simulink subsystem "CantileverCartesianRobotSubsystem"  (R2024a)
settings: Solver=VariableStepAuto  StartTime=0.0  StopTime=10.0  RelTol=1e-3
model mask{DOF=3DOF, configAxis=XYZ, heightColumn=0.4, widthColumn=0.05, positionColumn1=[-0.5,-0.5,0], positionColumn2=[0.5,-0.5,0], systemGuideX=Rail-block, strokeXMax=1, widthGuideX=0.05, diaScrewX=0.05, widthXMount=0.1, typeInertiaGuideX=Calculate from Geometry, densityGuideX=2700, massGuideX=0.1, COMGuideX=[0 0 0], MOIGuideX=[0.01 0.01 0.01], POIGuideX=[0 0 0], typeInertiaCarriageX=Calculate from Geometry, densityCarriageX=2700, massCarriageX=0.1, COMCarriageX=[0 0 0], MOICarriageX=[0.01 0.01 0.01], POICarriageX=[0 0 0], colorGuideX=[0.7 0.6 0.4], colorCarriageX=[0.5 0.5 0.9], systemGuideY=Rail-block, strokeYMax=1, widthGuideY=0.05, diaScrewY=0.05, widthYMount=0.05, typeInertiaGuideY=Calculate from Geometry, densityGuideY=2700, massGuideY=0.1, COMGuideY=[0 0 0], MOIGuideY=[0.01 0.01 0.01], POIGuideY=[0 0 0], typeInertiaCarriageY=Calculate from Geometry, densityCarriageY=2700, massCarriageY=0.1, COMCarriageY=[0 0 0], MOICarriageY=[0.01 0.01 0.01], POICarriageY=[0 0 0], colorGuideY=[0.7 0.6 0.4], colorCarriageY=[0.5 0.5 0.9], systemGuideZ=Rail-block, strokeZMax=1, widthGuideZ=0.05, diaScrewZ=0.05, shiftZAxisDown=015, widthZMount=0.05, typeInertiaGuideZ=Calculate from Geometry, densityGuideZ=2700, massGuideZ=0.1, COMGuideZ=[0 0 0], MOIGuideZ=[0.01 0.01 0.01], POIGuideZ=[0 0 0], typeInertiaCarriageZ=Calculate from Geometry, densityCarriageZ=2700, massCarriageZ=0.1, COMCarriageZ=[0 0 0], MOICarriageZ=[0.01 0.01 0.01], POICarriageZ=[0 0 0], colorGuideZ=[0.7 0.6 0.4], colorCarriageZ=[0.5 0.5 0.9]}
  mask prompts: DOF "Degrees of freedom"; configAxis "Axis configurations"; heightColumn "Column height (m)"; widthColumn "Column width (m)"; positionColumn1 "Column 1 position (m)"; positionColumn2 "Column 2 position (m)"; systemGuideX "Guide system"; strokeXMax "Maximum stroke (m)"; widthGuideX "Guide width (m)"; diaScrewX "Screw diameter (m)"; widthXMount "Mount width (m)"; typeInertiaGuideX "Inertia type"; densityGuideX "Density (kg/m^3)"; massGuideX "Mass (kg)"; COMGuideX "Center of mass (m)"; MOIGuideX "Moments of inertia (kg*m^2)"; POIGuideX "Products of inertia (kg*m^2)"; typeInertiaCarriageX "Inertia type"; densityCarriageX "Density (kg/m^3)"; massCarriageX "Mass (kg)"; COMCarriageX "Center of mass (m)"; MOICarriageX "Moments of inertia (kg*m^2)"; POICarriageX "Products of inertia (kg*m^2)"; colorGuideX "Linear guide color"; colorCarriageX "Carriage color"; systemGuideY "Guide system"; strokeYMax "Maximum stroke (m)"; widthGuideY "Guide width (m)"; diaScrewY "Screw diameter (m)"; widthYMount "Mount width (m)"; typeInertiaGuideY "Inertia type"; densityGuideY "Density (kg/m^3)"; massGuideY "Mass (kg)"; COMGuideY "Center of mass (m)"; MOIGuideY "Moments of inertia (kg*m^2)"; POIGuideY "Products of inertia (kg*m^2)"; typeInertiaCarriageY "Inertia type"; densityCarriageY "Density (kg/m^3)"; massCarriageY "Mass (kg)"; COMCarriageY "Center of mass (m)"; MOICarriageY "Moments of inertia (kg*m^2)"; POICarriageY "Products of inertia (kg*m^2)"; colorGuideY "Linear guide color"; colorCarriageY "Carriage color"; systemGuideZ "Guide system"; strokeZMax "Maximum stroke (m)"; widthGuideZ "Guide width (m)"; diaScrewZ "Screw diameter (m)"; shiftZAxisDown "Downward shift of Z-axis (m)"; widthZMount "Mount width (m)"; typeInertiaGuideZ "Inertia type"; densityGuideZ "Density (kg/m^3)"; massGuideZ "Mass (kg)"; COMGuideZ "Center of mass (m)"; MOIGuideZ "Moments of inertia (kg*m^2)"; POIGuideZ "Products of inertia (kg*m^2)"; typeInertiaCarriageZ "Inertia type"; densityCarriageZ "Density (kg/m^3)"; massCarriageZ "Mass (kg)"; COMCarriageZ "Center of mass (m)"; MOICarriageZ "Moments of inertia (kg*m^2)"; POICarriageZ "Products of inertia (kg*m^2)"; colorGuideZ "Linear guide color"; colorCarriageZ "Carriage color"
undefined symbols (not defined in the file): CartesianRobot, X, Y, Z
libraries: sm_lib x99, CartesianLib x44, nesl_utility x41
(part 2 of 4)

== system CantileverCartesianRobotSubsystem/CantileverCartesianRobotVariant/XY Cartesian/Structure1 ==
  Column1 : CartesianLib/Column  lengthColumn=heightColumn  widthColumn=widthColumn  typeInertiaColumn=Calculate from Geometry  densityColumn=7780  massColumn=1  CMColumn=[0 0 0]  MOIColumn=[1 1 1]  POIColumn=[0 0 0]  colorColumn=[0.8 0.2 0.2]
  Column2 : CartesianLib/Column  lengthColumn=heightColumn  widthColumn=widthColumn  typeInertiaColumn=Calculate from Geometry  densityColumn=7780  massColumn=1  CMColumn=[0 0 0]  MOIColumn=[1 1 1]  POIColumn=[0 0 0]  colorColumn=[0.8 0.2 0.2]
  Rigid Transform1 : sm_lib/Frames and Transforms/Rigid Transform  RotationMethod=None  FollAlignAxisA=+X  BaseAlignAxisA=+Y  FollAlignAxisB=+Y  BaseAlignAxisB=+Z  RotationStandardAxis=+Z  RotationAngle=0  RotationAngleUnits=deg  RotationArbitraryAxis=[0 0 1]  RotationSequenceAxes=FollowerAxes  RotationSequence=XYX  RotationSequenceAngles=[0 0 0]  RotationSequenceAnglesUnits=deg  RotationMatrix=[1 0 0;0 1 0;0 0 1]  Quaternion=[1 0 0 0]  TranslationMethod=Cartesian  TranslationCartesianOffset=positionColumn1  TranslationCartesianOffsetUnits=m  TranslationStandardAxis=+Z  TranslationStandardOffset=0  TranslationStandardOffsetUnits=m  TranslationROffset=0  TranslationROffsetUnits=m  TranslationThetaOffset=0  TranslationThetaOffsetUnits=deg  TranslationZOffset=0  TranslationZOffsetUnits=m
  Rigid Transform2 : sm_lib/Frames and Transforms/Rigid Transform  RotationMethod=None  FollAlignAxisA=+X  BaseAlignAxisA=+Y  FollAlignAxisB=+Y  BaseAlignAxisB=+Z  RotationStandardAxis=+Z  RotationAngle=0  RotationAngleUnits=deg  RotationArbitraryAxis=[0 0 1]  RotationSequenceAxes=FollowerAxes  RotationSequence=XYX  RotationSequenceAngles=[0 0 0]  RotationSequenceAnglesUnits=deg  RotationMatrix=[1 0 0;0 1 0;0 0 1]  Quaternion=[1 0 0 0]  TranslationMethod=Cartesian  TranslationCartesianOffset=positionColumn2  TranslationCartesianOffsetUnits=m  TranslationStandardAxis=+Z  TranslationStandardOffset=0  TranslationStandardOffsetUnits=m  TranslationROffset=0  TranslationROffsetUnits=m  TranslationThetaOffset=0  TranslationThetaOffsetUnits=deg  TranslationZOffset=0  TranslationZOffsetUnits=m
  Weld Joint : sm_lib/Joints/Weld Joint  JointMode=Normal  CompositeWrenchDir=FollowerOnBase  CompositeWrenchFrame=BaseFrame  SenseConstraintForce=off  SenseConstraintTorque=off  SenseTotalForce=off  SenseTotalTorque=off
  Weld Joint1 : sm_lib/Joints/Weld Joint  JointMode=Normal  CompositeWrenchDir=FollowerOnBase  CompositeWrenchFrame=BaseFrame  SenseConstraintForce=off  SenseConstraintTorque=off  SenseTotalForce=off  SenseTotalTorque=off
  XMount1 : CartesianLib/Mount  typeMount=Plate mount  widthMount=widthXMount  angleMount=45  angleRotate=0  typeInertiaMount=Calculate from Geometry  densityMount=7780  massMount=0.1  CMMount=[0 0 0]  MOIMount=[1 1 1]  POIMount=[0 0 0]  colorMount=[0.35 0.25 0.25]
  XMount2 : CartesianLib/Mount  typeMount=Plate mount  widthMount=widthXMount  angleMount=45  angleRotate=0  typeInertiaMount=Calculate from Geometry  densityMount=7780  massMount=0.1  CMMount=[0 0 0]  MOIMount=[1 1 1]  POIMount=[0 0 0]  colorMount=[0.35 0.25 0.25]
  F1 : PMIOPort  Side=Left
  B : PMIOPort  Port=2  Side=Right
  F2 : PMIOPort  Port=3  Side=Left
  connections:
  Weld Joint1/RConn1 -- Column2/RConn1
  Rigid Transform1/RConn1 -- Weld Joint/LConn1
  Rigid Transform2/RConn1 -- Weld Joint1/LConn1
  B/RConn1 -- Rigid Transform2/LConn1 -- Rigid Transform1/LConn1
  F2/RConn1 -- XMount2/LConn1
  XMount2/RConn1 -- Column2/LConn1
  Column1/LConn1 -- XMount1/RConn1
  XMount1/LConn1 -- F1/RConn1
  Weld Joint/RConn1 -- Column1/RConn1

== system CantileverCartesianRobotSubsystem/CantileverCartesianRobotVariant/XY Cartesian/Subsystem ==
  note: Dummy ZS signals
  Constant : Constant  Value=0
  Constant1 : Constant  Value=0
  Constant2 : Constant  Value=0
  Bus Element Out : Outport  PortName=ZS  Element=Zp (m)
  BusElementOut : Outport  PortName=ZS  Element=Zv (m/s)
  BusElementOut1 : Outport  PortName=ZS  Element=Za (m^2/s)
  wires:
  Constant/1 -> Bus Element Out/1
  Constant1/1 -> BusElementOut/1
  Constant2/1 -> BusElementOut1/1

== system CantileverCartesianRobotSubsystem/CantileverCartesianRobotVariant/XY Cartesian/Subsystem1 ==
  note: Dummy RS signals
  Constant : Constant  Value=0
  Constant1 : Constant  Value=0
  Bus Element Out : Outport  PortName=RS  Element=q (rad)
  BusElementOut : Outport  PortName=RS  Element=w (rad/s)
  wires:
  Constant/1 -> Bus Element Out/1
  Constant1/1 -> BusElementOut/1

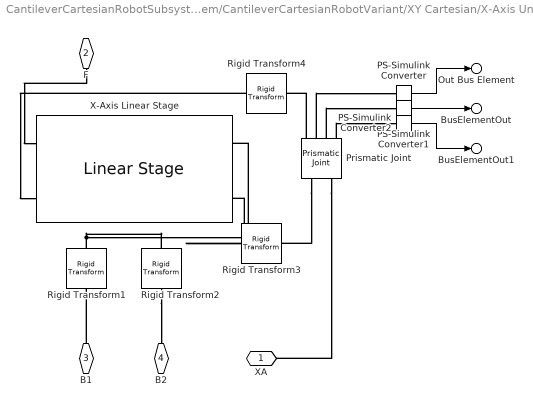
== system CantileverCartesianRobotSubsystem/CantileverCartesianRobotVariant/XY Cartesian/X-Axis Unit ==
  PS-Simulink Converter : nesl_utility/PS-Simulink Converter  PhysicalDomain=network_engine_domain  SubClassName=ps_output  LeftPortType=input  RightPortType=output  PseudoPeriodic=off  Frequencies=[]  VectorFormat=inherit  Unit=inherit  AffineConversion=off
  PS-Simulink Converter1 : nesl_utility/PS-Simulink Converter  PhysicalDomain=network_engine_domain  SubClassName=ps_output  LeftPortType=input  RightPortType=output  PseudoPeriodic=off  Frequencies=[]  VectorFormat=inherit  Unit=inherit  AffineConversion=off
  PS-Simulink Converter2 : nesl_utility/PS-Simulink Converter  PhysicalDomain=network_engine_domain  SubClassName=ps_output  LeftPortType=input  RightPortType=output  PseudoPeriodic=off  Frequencies=[]  VectorFormat=inherit  Unit=inherit  AffineConversion=off
  Prismatic Joint : sm_lib/Joints/Prismatic Joint  JointMode=Normal  CompositeWrenchDir=FollowerOnBase  CompositeWrenchFrame=BaseFrame  SenseConstraintForce=off  SenseConstraintTorque=off  SenseTotalForce=off  SenseTotalTorque=off  PositionTargetSpecify=off  PositionTargetPriority=High  PositionTargetValue=0  PositionTargetValueUnits=m  VelocityTargetSpecify=off  VelocityTargetPriority=High  VelocityTargetValue=0  VelocityTargetValueUnits=m/s  EquilibriumPosition=0  EquilibriumPositionUnits=m  SpringStiffness=0  SpringStiffnessUnits=N/m  DampingCoefficient=0  DampingCoefficientUnits=N/(m/s)  LowerLimitSpecify=on  LowerLimitBound=-0.5*strokeXMax  LowerLimitBoundUnits=m  LowerLimitStiffness=1e6  LowerLimitStiffnessUnits=N/m  LowerLimitDamping=1e3  LowerLimitDampingUnits=N/(m/s)  LowerLimitTransitionRegionWidth=1e-4  LowerLimitTransitionRegionWidthUnits=m  UpperLimitSpecify=on  UpperLimitBound=0.5*strokeXMax  UpperLimitBoundUnits=m  UpperLimitStiffness=1e6  UpperLimitStiffnessUnits=N/m  UpperLimitDamping=1e3  UpperLimitDampingUnits=N/(m/s)  UpperLimitTransitionRegionWidth=1e-4  UpperLimitTransitionRegionWidthUnits=m  TorqueActuationMode=InputTorque  MotionActuationMode=ComputedMotion  SensePosition=on  SenseVelocity=on  SenseAcceleration=on  SenseTorqueForce=off  SenseLowerLimitTorqueForce=off  SenseUpperLimitTorqueForce=off
  Rigid Transform1 : sm_lib/Frames and Transforms/Rigid Transform  RotationMethod=None  FollAlignAxisA=+X  BaseAlignAxisA=+Y  FollAlignAxisB=+Y  BaseAlignAxisB=+Z  RotationStandardAxis=+Z  RotationAngle=0  RotationAngleUnits=deg  RotationArbitraryAxis=[0 0 1]  RotationSequenceAxes=FollowerAxes  RotationSequence=XYX  RotationSequenceAngles=[0 0 0]  RotationSequenceAnglesUnits=deg  RotationMatrix=[1 0 0;0 1 0;0 0 1]  Quaternion=[1 0 0 0]  TranslationMethod=StandardAxis  TranslationCartesianOffset=[-positionColumn1(1) 0 0]  TranslationCartesianOffsetUnits=m  TranslationStandardAxis=+X  TranslationStandardOffset=-positionColumn1(1)  TranslationStandardOffsetUnits=m  TranslationROffset=0  TranslationROffsetUnits=m  TranslationThetaOffset=0  TranslationThetaOffsetUnits=deg  TranslationZOffset=0  TranslationZOffsetUnits=m
  Rigid Transform2 : sm_lib/Frames and Transforms/Rigid Transform  RotationMethod=None  FollAlignAxisA=+X  BaseAlignAxisA=+Y  FollAlignAxisB=+Y  BaseAlignAxisB=+Z  RotationStandardAxis=+Z  RotationAngle=0  RotationAngleUnits=deg  RotationArbitraryAxis=[0 0 1]  RotationSequenceAxes=FollowerAxes  RotationSequence=XYX  RotationSequenceAngles=[0 0 0]  RotationSequenceAnglesUnits=deg  RotationMatrix=[1 0 0;0 1 0;0 0 1]  Quaternion=[1 0 0 0]  TranslationMethod=StandardAxis  TranslationCartesianOffset=[-positionColumn2(1) 0 0]  TranslationCartesianOffsetUnits=m  TranslationStandardAxis=+X  TranslationStandardOffset=-positionColumn2(1)  TranslationStandardOffsetUnits=m  TranslationROffset=0  TranslationROffsetUnits=m  TranslationThetaOffset=0  TranslationThetaOffsetUnits=deg  TranslationZOffset=0  TranslationZOffsetUnits=m
  Rigid Transform3 : sm_lib/Frames and Transforms/Rigid Transform  RotationMethod=StandardAxis  FollAlignAxisA=+X  BaseAlignAxisA=+Y  FollAlignAxisB=+Y  BaseAlignAxisB=+Z  RotationStandardAxis=+Y  RotationAngle=90  RotationAngleUnits=deg  RotationArbitraryAxis=[0 0 1]  RotationSequenceAxes=FollowerAxes  RotationSequence=XYX  RotationSequenceAngles=[0 0 0]  RotationSequenceAnglesUnits=deg  RotationMatrix=[1 0 0;0 1 0;0 0 1]  Quaternion=[1 0 0 0]  TranslationMethod=None  TranslationCartesianOffset=[0 0 0]  TranslationCartesianOffsetUnits=m  TranslationStandardAxis=+Z  TranslationStandardOffset=0  TranslationStandardOffsetUnits=m  TranslationROffset=0  TranslationROffsetUnits=m  TranslationThetaOffset=0  TranslationThetaOffsetUnits=deg  TranslationZOffset=0  TranslationZOffsetUnits=m
  Rigid Transform4 : sm_lib/Frames and Transforms/Rigid Transform  RotationMethod=StandardAxis  FollAlignAxisA=+X  BaseAlignAxisA=+Y  FollAlignAxisB=+Y  BaseAlignAxisB=+Z  RotationStandardAxis=+Y  RotationAngle=-90  RotationAngleUnits=deg  RotationArbitraryAxis=[0 0 1]  RotationSequenceAxes=FollowerAxes  RotationSequence=XYX  RotationSequenceAngles=[0 0 0]  RotationSequenceAnglesUnits=deg  RotationMatrix=[1 0 0;0 1 0;0 0 1]  Quaternion=[1 0 0 0]  TranslationMethod=None  TranslationCartesianOffset=[0 0 0]  TranslationCartesianOffsetUnits=m  TranslationStandardAxis=+Z  TranslationStandardOffset=0  TranslationStandardOffsetUnits=m  TranslationROffset=0  TranslationROffsetUnits=m  TranslationThetaOffset=0  TranslationThetaOffsetUnits=deg  TranslationZOffset=0  TranslationZOffsetUnits=m
  X-Axis Linear Stage : CartesianLib/Linear Stage  systemGuide=Rail-block  axisGuide=X-axis  stroke=1  widthRail=0.05  diaScrew=0.05  typeInertiaGuide=Calculate from Geometry  densityGuide=2700  massGuide=0.1  CMGuide=[0 0 0]  MOIGuide=[0.01 0.01 0.01]  POIGuide=[0 0 0]  typeInertiaCarriage=Calculate from Geometry  densityCarriage=2700  massCarriage=0.1  CMCarriage=[0 0 0]  MOICarriage=[0.01 0.01 0.01]  POICarriage=[0 0 0]  colorGuide=colorGuideX  colorCarriage=colorCarriageX
  XA : PMIOPort  Side=Left
  F : PMIOPort  Port=2  Side=Left
  B1 : PMIOPort  Port=3  Side=Right
  B2 : PMIOPort  Port=4  Side=Right
  Out Bus Element : Outport  PortName=XS  Element=Xp (m)
  BusElementOut : Outport  PortName=XS  Element=Xv (m/s)
  BusElementOut1 : Outport  PortName=XS  Element=Xa (m^2/s)
  wires:
  PS-Simulink Converter2/1 -> BusElementOut1/1
  PS-Simulink Converter1/1 -> BusElementOut/1
  PS-Simulink Converter/1 -> Out Bus Element/1
  connections:
  Prismatic Joint/RConn4 -- PS-Simulink Converter2/LConn1
  Prismatic Joint/RConn3 -- PS-Simulink Converter1/LConn1
  Prismatic Joint/RConn2 -- PS-Simulink Converter/LConn1
  Rigid Transform2/LConn1 -- B2/RConn1
  Rigid Transform3/LConn1 -- X-Axis Linear Stage/RConn2
  X-Axis Linear Stage/RConn1 -- Rigid Transform2/RConn1 -- Rigid Transform1/RConn1
  Prismatic Joint/LConn1 -- Rigid Transform3/RConn1
  F/RConn1 -- X-Axis Linear Stage/LConn1
  Prismatic Joint/RConn1 -- Rigid Transform4/LConn1
  B1/RConn1 -- Rigid Transform1/LConn1
  Prismatic Joint/LConn2 -- XA/RConn1
  Rigid Transform4/RConn1 -- X-Axis Linear Stage/LConn2

== system CantileverCartesianRobotSubsystem/CantileverCartesianRobotVariant/XY Cartesian/Y-Axis Unit ==
  PS-Simulink Converter : nesl_utility/PS-Simulink Converter  PhysicalDomain=network_engine_domain  SubClassName=ps_output  LeftPortType=input  RightPortType=output  PseudoPeriodic=off  Frequencies=[]  VectorFormat=inherit  Unit=inherit  AffineConversion=off
  PS-Simulink Converter1 : nesl_utility/PS-Simulink Converter  PhysicalDomain=network_engine_domain  SubClassName=ps_output  LeftPortType=input  RightPortType=output  PseudoPeriodic=off  Frequencies=[]  VectorFormat=inherit  Unit=inherit  AffineConversion=off
  PS-Simulink Converter2 : nesl_utility/PS-Simulink Converter  PhysicalDomain=network_engine_domain  SubClassName=ps_output  LeftPortType=input  RightPortType=output  PseudoPeriodic=off  Frequencies=[]  VectorFormat=inherit  Unit=inherit  AffineConversion=off
  Prismatic Joint2 : sm_lib/Joints/Prismatic Joint  JointMode=Normal  CompositeWrenchDir=FollowerOnBase  CompositeWrenchFrame=BaseFrame  SenseConstraintForce=off  SenseConstraintTorque=off  SenseTotalForce=off  SenseTotalTorque=off  PositionTargetSpecify=off  PositionTargetPriority=High  PositionTargetValue=0  PositionTargetValueUnits=m  VelocityTargetSpecify=off  VelocityTargetPriority=High  VelocityTargetValue=0  VelocityTargetValueUnits=m/s  EquilibriumPosition=0  EquilibriumPositionUnits=m  SpringStiffness=0  SpringStiffnessUnits=N/m  DampingCoefficient=0  DampingCoefficientUnits=N/(m/s)  LowerLimitSpecify=on  LowerLimitBound=-0.5*strokeYMax  LowerLimitBoundUnits=m  LowerLimitStiffness=1e6  LowerLimitStiffnessUnits=N/m  LowerLimitDamping=1e3  LowerLimitDampingUnits=N/(m/s)  LowerLimitTransitionRegionWidth=1e-4  LowerLimitTransitionRegionWidthUnits=m  UpperLimitSpecify=on  UpperLimitBound=0.5*strokeYMax  UpperLimitBoundUnits=m  UpperLimitStiffness=1e6  UpperLimitStiffnessUnits=N/m  UpperLimitDamping=1e3  UpperLimitDampingUnits=N/(m/s)  UpperLimitTransitionRegionWidth=1e-4  UpperLimitTransitionRegionWidthUnits=m  TorqueActuationMode=InputTorque  MotionActuationMode=ComputedMotion  SensePosition=on  SenseVelocity=on  SenseAcceleration=on  SenseTorqueForce=off  SenseLowerLimitTorqueForce=off  SenseUpperLimitTorqueForce=off
  Rigid Transform1 : sm_lib/Frames and Transforms/Rigid Transform  RotationMethod=None  FollAlignAxisA=+X  BaseAlignAxisA=+Y  FollAlignAxisB=+Y  BaseAlignAxisB=+Z  RotationStandardAxis=+Z  RotationAngle=0  RotationAngleUnits=deg  RotationArbitraryAxis=[0 0 1]  RotationSequenceAxes=BaseAxes  RotationSequence=XYZ  RotationSequenceAngles=[0 0 0]  RotationSequenceAnglesUnits=deg  RotationMatrix=[1 0 0;0 1 0;0 0 1]  Quaternion=[1 0 0 0]  TranslationMethod=StandardAxis  TranslationCartesianOffset=[0 0 0]  TranslationCartesianOffsetUnits=m  TranslationStandardAxis=+Y  TranslationStandardOffset=-positionColumn1(2)  TranslationStandardOffsetUnits=m  TranslationROffset=0  TranslationROffsetUnits=m  TranslationThetaOffset=0  TranslationThetaOffsetUnits=deg  TranslationZOffset=0  TranslationZOffsetUnits=m
  Rigid Transform3 : sm_lib/Frames and Transforms/Rigid Transform  RotationMethod=StandardAxis  FollAlignAxisA=+X  BaseAlignAxisA=+Y  FollAlignAxisB=+Y  BaseAlignAxisB=+Z  RotationStandardAxis=+X  RotationAngle=-90  RotationAngleUnits=deg  RotationArbitraryAxis=[0 0 1]  RotationSequenceAxes=FollowerAxes  RotationSequence=XYX  RotationSequenceAngles=[0 0 0]  RotationSequenceAnglesUnits=deg  RotationMatrix=[1 0 0;0 1 0;0 0 1]  Quaternion=[1 0 0 0]  TranslationMethod=None  TranslationCartesianOffset=[0 0 0]  TranslationCartesianOffsetUnits=m  TranslationStandardAxis=+Z  TranslationStandardOffset=0  TranslationStandardOffsetUnits=m  TranslationROffset=0  TranslationROffsetUnits=m  TranslationThetaOffset=0  TranslationThetaOffsetUnits=deg  TranslationZOffset=0  TranslationZOffsetUnits=m
  Rigid Transform4 : sm_lib/Frames and Transforms/Rigid Transform  RotationMethod=StandardAxis  FollAlignAxisA=+X  BaseAlignAxisA=+Y  FollAlignAxisB=+Y  BaseAlignAxisB=+Z  RotationStandardAxis=+X  RotationAngle=90  RotationAngleUnits=deg  RotationArbitraryAxis=[0 0 1]  RotationSequenceAxes=FollowerAxes  RotationSequence=XYX  RotationSequenceAngles=[0 0 0]  RotationSequenceAnglesUnits=deg  RotationMatrix=[1 0 0;0 1 0;0 0 1]  Quaternion=[1 0 0 0]  TranslationMethod=None  TranslationCartesianOffset=[0 0 0]  TranslationCartesianOffsetUnits=m  TranslationStandardAxis=+Z  TranslationStandardOffset=0  TranslationStandardOffsetUnits=m  TranslationROffset=0  TranslationROffsetUnits=m  TranslationThetaOffset=0  TranslationThetaOffsetUnits=deg  TranslationZOffset=0  TranslationZOffsetUnits=m
  Y-Axis Linear Stage : CartesianLib/Linear Stage  systemGuide=Rail-block  axisGuide=Y-axis  stroke=1  widthRail=0.05  diaScrew=0.05  typeInertiaGuide=Calculate from Geometry  densityGuide=2700  massGuide=0.1  CMGuide=[0 0 0]  MOIGuide=[0.01 0.01 0.01]  POIGuide=[0 0 0]  typeInertiaCarriage=Calculate from Geometry  densityCarriage=2700  massCarriage=0.1  CMCarriage=[0 0 0]  MOICarriage=[0.01 0.01 0.01]  POICarriage=[0 0 0]  colorGuide=colorGuideY  colorCarriage=colorCarriageY
  YA : PMIOPort  Side=Left
  F : PMIOPort  Port=2  Side=Left
  B : PMIOPort  Port=3  Side=Right
  Out Bus Element : Outport  PortName=YS  Element=Yp (m)
  BusElementOut : Outport  PortName=YS  Element=Yv (m/s)
  BusElementOut1 : Outport  PortName=YS  Element=Ya (m^2/s)
  wires:
  PS-Simulink Converter2/1 -> BusElementOut1/1
  PS-Simulink Converter1/1 -> BusElementOut/1
  PS-Simulink Converter/1 -> Out Bus Element/1
  connections:
  Prismatic Joint2/RConn2 -- PS-Simulink Converter/LConn1
  PS-Simulink Converter2/LConn1 -- Prismatic Joint2/RConn4
  Prismatic Joint2/RConn3 -- PS-Simulink Converter1/LConn1
  F/RConn1 -- Y-Axis Linear Stage/LConn1
  Rigid Transform1/LConn1 -- B/RConn1
  Prismatic Joint2/LConn2 -- YA/RConn1
  Rigid Transform1/RConn1 -- Y-Axis Linear Stage/RConn1
  Prismatic Joint2/RConn1 -- Rigid Transform4/LConn1
  Rigid Transform3/LConn1 -- Y-Axis Linear Stage/RConn2
  Rigid Transform4/RConn1 -- Y-Axis Linear Stage/LConn2
  Prismatic Joint2/LConn1 -- Rigid Transform3/RConn1

== system CantileverCartesianRobotSubsystem/CantileverCartesianRobotVariant/XYZ Cartesian/Structure1 ==
  Column1 : CartesianLib/Column  lengthColumn=heightColumn  widthColumn=widthColumn  typeInertiaColumn=Calculate from Geometry  densityColumn=7780  massColumn=1  CMColumn=[0 0 0]  MOIColumn=[1 1 1]  POIColumn=[0 0 0]  colorColumn=[0.8 0.2 0.2]
  Column2 : CartesianLib/Column  lengthColumn=heightColumn  widthColumn=widthColumn  typeInertiaColumn=Calculate from Geometry  densityColumn=7780  massColumn=1  CMColumn=[0 0 0]  MOIColumn=[1 1 1]  POIColumn=[0 0 0]  colorColumn=[0.8 0.2 0.2]
  Rigid Transform1 : sm_lib/Frames and Transforms/Rigid Transform  RotationMethod=None  FollAlignAxisA=+X  BaseAlignAxisA=+Y  FollAlignAxisB=+Y  BaseAlignAxisB=+Z  RotationStandardAxis=+Z  RotationAngle=0  RotationAngleUnits=deg  RotationArbitraryAxis=[0 0 1]  RotationSequenceAxes=FollowerAxes  RotationSequence=XYX  RotationSequenceAngles=[0 0 0]  RotationSequenceAnglesUnits=deg  RotationMatrix=[1 0 0;0 1 0;0 0 1]  Quaternion=[1 0 0 0]  TranslationMethod=Cartesian  TranslationCartesianOffset=positionColumn1  TranslationCartesianOffsetUnits=m  TranslationStandardAxis=+Z  TranslationStandardOffset=0  TranslationStandardOffsetUnits=m  TranslationROffset=0  TranslationROffsetUnits=m  TranslationThetaOffset=0  TranslationThetaOffsetUnits=deg  TranslationZOffset=0  TranslationZOffsetUnits=m
  Rigid Transform2 : sm_lib/Frames and Transforms/Rigid Transform  RotationMethod=None  FollAlignAxisA=+X  BaseAlignAxisA=+Y  FollAlignAxisB=+Y  BaseAlignAxisB=+Z  RotationStandardAxis=+Z  RotationAngle=0  RotationAngleUnits=deg  RotationArbitraryAxis=[0 0 1]  RotationSequenceAxes=FollowerAxes  RotationSequence=XYX  RotationSequenceAngles=[0 0 0]  RotationSequenceAnglesUnits=deg  RotationMatrix=[1 0 0;0 1 0;0 0 1]  Quaternion=[1 0 0 0]  TranslationMethod=Cartesian  TranslationCartesianOffset=positionColumn2  TranslationCartesianOffsetUnits=m  TranslationStandardAxis=+Z  TranslationStandardOffset=0  TranslationStandardOffsetUnits=m  TranslationROffset=0  TranslationROffsetUnits=m  TranslationThetaOffset=0  TranslationThetaOffsetUnits=deg  TranslationZOffset=0  TranslationZOffsetUnits=m
  Weld Joint : sm_lib/Joints/Weld Joint  JointMode=Normal  CompositeWrenchDir=FollowerOnBase  CompositeWrenchFrame=BaseFrame  SenseConstraintForce=off  SenseConstraintTorque=off  SenseTotalForce=off  SenseTotalTorque=off
  Weld Joint1 : sm_lib/Joints/Weld Joint  JointMode=Normal  CompositeWrenchDir=FollowerOnBase  CompositeWrenchFrame=BaseFrame  SenseConstraintForce=off  SenseConstraintTorque=off  SenseTotalForce=off  SenseTotalTorque=off
  XMount1 : CartesianLib/Mount  typeMount=Plate mount  widthMount=widthXMount  angleMount=45  angleRotate=0  typeInertiaMount=Calculate from Geometry  densityMount=7780  massMount=0.1  CMMount=[0 0 0]  MOIMount=[1 1 1]  POIMount=[0 0 0]  colorMount=[0.35 0.25 0.25]
  XMount2 : CartesianLib/Mount  typeMount=Plate mount  widthMount=widthXMount  angleMount=45  angleRotate=0  typeInertiaMount=Calculate from Geometry  densityMount=7780  massMount=0.1  CMMount=[0 0 0]  MOIMount=[1 1 1]  POIMount=[0 0 0]  colorMount=[0.35 0.25 0.25]
  F1 : PMIOPort  Side=Left
  B : PMIOPort  Port=2  Side=Right
  F2 : PMIOPort  Port=3  Side=Left
  connections:
  Weld Joint1/RConn1 -- Column2/RConn1
  Rigid Transform2/RConn1 -- Weld Joint1/LConn1
  Rigid Transform1/RConn1 -- Weld Joint/LConn1
  F2/RConn1 -- XMount2/LConn1
  Rigid Transform1/LConn1 -- B/RConn1 -- Rigid Transform2/LConn1
  XMount2/RConn1 -- Column2/LConn1
  Column1/LConn1 -- XMount1/RConn1
  XMount1/LConn1 -- F1/RConn1
  Weld Joint/RConn1 -- Column1/RConn1

== system CantileverCartesianRobotSubsystem/CantileverCartesianRobotVariant/XYZ Cartesian/Subsystem1 ==
  note: Dummy RS signals
  Constant : Constant  Value=0
  Constant1 : Constant  Value=0
  Bus Element Out : Outport  PortName=RS  Element=q (rad)
  BusElementOut : Outport  PortName=RS  Element=w (rad/s)
  wires:
  Constant/1 -> Bus Element Out/1
  Constant1/1 -> BusElementOut/1

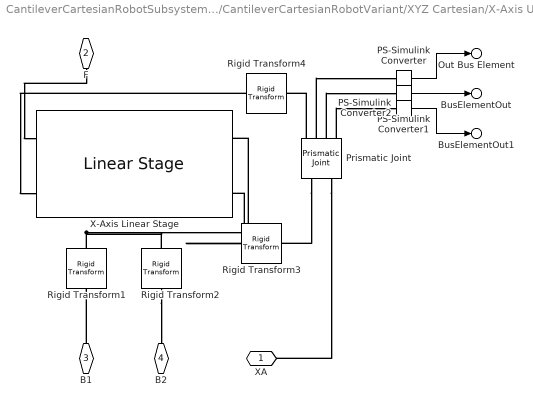
== system CantileverCartesianRobotSubsystem/CantileverCartesianRobotVariant/XYZ Cartesian/X-Axis Unit ==
  PS-Simulink Converter : nesl_utility/PS-Simulink Converter  PhysicalDomain=network_engine_domain  SubClassName=ps_output  LeftPortType=input  RightPortType=output  PseudoPeriodic=off  Frequencies=[]  VectorFormat=inherit  Unit=inherit  AffineConversion=off
  PS-Simulink Converter1 : nesl_utility/PS-Simulink Converter  PhysicalDomain=network_engine_domain  SubClassName=ps_output  LeftPortType=input  RightPortType=output  PseudoPeriodic=off  Frequencies=[]  VectorFormat=inherit  Unit=inherit  AffineConversion=off
  PS-Simulink Converter2 : nesl_utility/PS-Simulink Converter  PhysicalDomain=network_engine_domain  SubClassName=ps_output  LeftPortType=input  RightPortType=output  PseudoPeriodic=off  Frequencies=[]  VectorFormat=inherit  Unit=inherit  AffineConversion=off
  Prismatic Joint : sm_lib/Joints/Prismatic Joint  JointMode=Normal  CompositeWrenchDir=FollowerOnBase  CompositeWrenchFrame=BaseFrame  SenseConstraintForce=off  SenseConstraintTorque=off  SenseTotalForce=off  SenseTotalTorque=off  PositionTargetSpecify=off  PositionTargetPriority=High  PositionTargetValue=0  PositionTargetValueUnits=m  VelocityTargetSpecify=off  VelocityTargetPriority=High  VelocityTargetValue=0  VelocityTargetValueUnits=m/s  EquilibriumPosition=0  EquilibriumPositionUnits=m  SpringStiffness=0  SpringStiffnessUnits=N/m  DampingCoefficient=0  DampingCoefficientUnits=N/(m/s)  LowerLimitSpecify=on  LowerLimitBound=-0.5*strokeXMax  LowerLimitBoundUnits=m  LowerLimitStiffness=1e6  LowerLimitStiffnessUnits=N/m  LowerLimitDamping=1e3  LowerLimitDampingUnits=N/(m/s)  LowerLimitTransitionRegionWidth=1e-4  LowerLimitTransitionRegionWidthUnits=m  UpperLimitSpecify=on  UpperLimitBound=0.5*strokeXMax  UpperLimitBoundUnits=m  UpperLimitStiffness=1e6  UpperLimitStiffnessUnits=N/m  UpperLimitDamping=1e3  UpperLimitDampingUnits=N/(m/s)  UpperLimitTransitionRegionWidth=1e-4  UpperLimitTransitionRegionWidthUnits=m  TorqueActuationMode=InputTorque  MotionActuationMode=ComputedMotion  SensePosition=on  SenseVelocity=on  SenseAcceleration=on  SenseTorqueForce=off  SenseLowerLimitTorqueForce=off  SenseUpperLimitTorqueForce=off
  Rigid Transform1 : sm_lib/Frames and Transforms/Rigid Transform  RotationMethod=None  FollAlignAxisA=+X  BaseAlignAxisA=+Y  FollAlignAxisB=+Y  BaseAlignAxisB=+Z  RotationStandardAxis=+Z  RotationAngle=0  RotationAngleUnits=deg  RotationArbitraryAxis=[0 0 1]  RotationSequenceAxes=FollowerAxes  RotationSequence=XYX  RotationSequenceAngles=[0 0 0]  RotationSequenceAnglesUnits=deg  RotationMatrix=[1 0 0;0 1 0;0 0 1]  Quaternion=[1 0 0 0]  TranslationMethod=StandardAxis  TranslationCartesianOffset=[-positionColumn1(1) 0 0]  TranslationCartesianOffsetUnits=m  TranslationStandardAxis=+X  TranslationStandardOffset=-positionColumn1(1)  TranslationStandardOffsetUnits=m  TranslationROffset=0  TranslationROffsetUnits=m  TranslationThetaOffset=0  TranslationThetaOffsetUnits=deg  TranslationZOffset=0  TranslationZOffsetUnits=m
  Rigid Transform2 : sm_lib/Frames and Transforms/Rigid Transform  RotationMethod=None  FollAlignAxisA=+X  BaseAlignAxisA=+Y  FollAlignAxisB=+Y  BaseAlignAxisB=+Z  RotationStandardAxis=+Z  RotationAngle=0  RotationAngleUnits=deg  RotationArbitraryAxis=[0 0 1]  RotationSequenceAxes=FollowerAxes  RotationSequence=XYX  RotationSequenceAngles=[0 0 0]  RotationSequenceAnglesUnits=deg  RotationMatrix=[1 0 0;0 1 0;0 0 1]  Quaternion=[1 0 0 0]  TranslationMethod=StandardAxis  TranslationCartesianOffset=[-positionColumn2(1) 0 0]  TranslationCartesianOffsetUnits=m  TranslationStandardAxis=+X  TranslationStandardOffset=-positionColumn2(1)  TranslationStandardOffsetUnits=m  TranslationROffset=0  TranslationROffsetUnits=m  TranslationThetaOffset=0  TranslationThetaOffsetUnits=deg  TranslationZOffset=0  TranslationZOffsetUnits=m
  Rigid Transform3 : sm_lib/Frames and Transforms/Rigid Transform  RotationMethod=StandardAxis  FollAlignAxisA=+X  BaseAlignAxisA=+Y  FollAlignAxisB=+Y  BaseAlignAxisB=+Z  RotationStandardAxis=+Y  RotationAngle=90  RotationAngleUnits=deg  RotationArbitraryAxis=[0 0 1]  RotationSequenceAxes=FollowerAxes  RotationSequence=XYX  RotationSequenceAngles=[0 0 0]  RotationSequenceAnglesUnits=deg  RotationMatrix=[1 0 0;0 1 0;0 0 1]  Quaternion=[1 0 0 0]  TranslationMethod=None  TranslationCartesianOffset=[0 0 0]  TranslationCartesianOffsetUnits=m  TranslationStandardAxis=+Z  TranslationStandardOffset=0  TranslationStandardOffsetUnits=m  TranslationROffset=0  TranslationROffsetUnits=m  TranslationThetaOffset=0  TranslationThetaOffsetUnits=deg  TranslationZOffset=0  TranslationZOffsetUnits=m
  Rigid Transform4 : sm_lib/Frames and Transforms/Rigid Transform  RotationMethod=StandardAxis  FollAlignAxisA=+X  BaseAlignAxisA=+Y  FollAlignAxisB=+Y  BaseAlignAxisB=+Z  RotationStandardAxis=+Y  RotationAngle=-90  RotationAngleUnits=deg  RotationArbitraryAxis=[0 0 1]  RotationSequenceAxes=FollowerAxes  RotationSequence=XYX  RotationSequenceAngles=[0 0 0]  RotationSequenceAnglesUnits=deg  RotationMatrix=[1 0 0;0 1 0;0 0 1]  Quaternion=[1 0 0 0]  TranslationMethod=None  TranslationCartesianOffset=[0 0 0]  TranslationCartesianOffsetUnits=m  TranslationStandardAxis=+Z  TranslationStandardOffset=0  TranslationStandardOffsetUnits=m  TranslationROffset=0  TranslationROffsetUnits=m  TranslationThetaOffset=0  TranslationThetaOffsetUnits=deg  TranslationZOffset=0  TranslationZOffsetUnits=m
  X-Axis Linear Stage : CartesianLib/Linear Stage  systemGuide=Rail-block  axisGuide=X-axis  stroke=1  widthRail=0.05  diaScrew=0.05  typeInertiaGuide=Calculate from Geometry  densityGuide=2700  massGuide=0.1  CMGuide=[0 0 0]  MOIGuide=[0.01 0.01 0.01]  POIGuide=[0 0 0]  typeInertiaCarriage=Calculate from Geometry  densityCarriage=2700  massCarriage=0.1  CMCarriage=[0 0 0]  MOICarriage=[0.01 0.01 0.01]  POICarriage=[0 0 0]  colorGuide=colorGuideX  colorCarriage=colorCarriageX
  XA : PMIOPort  Side=Left
  F : PMIOPort  Port=2  Side=Left
  B1 : PMIOPort  Port=3  Side=Right
  B2 : PMIOPort  Port=4  Side=Right
  Out Bus Element : Outport  PortName=XS  Element=Xp (m)
  BusElementOut : Outport  PortName=XS  Element=Xv (m/s)
  BusElementOut1 : Outport  PortName=XS  Element=Xa (m^2/s)
  wires:
  PS-Simulink Converter1/1 -> BusElementOut/1
  PS-Simulink Converter2/1 -> BusElementOut1/1
  PS-Simulink Converter/1 -> Out Bus Element/1
  connections:
  Prismatic Joint/RConn2 -- PS-Simulink Converter/LConn1
  Prismatic Joint/RConn3 -- PS-Simulink Converter1/LConn1
  Prismatic Joint/RConn4 -- PS-Simulink Converter2/LConn1
  Rigid Transform2/LConn1 -- B2/RConn1
  Rigid Transform3/LConn1 -- X-Axis Linear Stage/RConn2
  X-Axis Linear Stage/RConn1 -- Rigid Transform1/RConn1 -- Rigid Transform2/RConn1
  Prismatic Joint/LConn1 -- Rigid Transform3/RConn1
  F/RConn1 -- X-Axis Linear Stage/LConn1
  Prismatic Joint/RConn1 -- Rigid Transform4/LConn1
  B1/RConn1 -- Rigid Transform1/LConn1
  Prismatic Joint/LConn2 -- XA/RConn1
  Rigid Transform4/RConn1 -- X-Axis Linear Stage/LConn2

== system CantileverCartesianRobotSubsystem/CantileverCartesianRobotVariant/XYZ Cartesian/Y-Axis Unit ==
  PS-Simulink Converter : nesl_utility/PS-Simulink Converter  PhysicalDomain=network_engine_domain  SubClassName=ps_output  LeftPortType=input  RightPortType=output  PseudoPeriodic=off  Frequencies=[]  VectorFormat=inherit  Unit=inherit  AffineConversion=off
  PS-Simulink Converter1 : nesl_utility/PS-Simulink Converter  PhysicalDomain=network_engine_domain  SubClassName=ps_output  LeftPortType=input  RightPortType=output  PseudoPeriodic=off  Frequencies=[]  VectorFormat=inherit  Unit=inherit  AffineConversion=off
  PS-Simulink Converter2 : nesl_utility/PS-Simulink Converter  PhysicalDomain=network_engine_domain  SubClassName=ps_output  LeftPortType=input  RightPortType=output  PseudoPeriodic=off  Frequencies=[]  VectorFormat=inherit  Unit=inherit  AffineConversion=off
  Prismatic Joint2 : sm_lib/Joints/Prismatic Joint  JointMode=Normal  CompositeWrenchDir=FollowerOnBase  CompositeWrenchFrame=BaseFrame  SenseConstraintForce=off  SenseConstraintTorque=off  SenseTotalForce=off  SenseTotalTorque=off  PositionTargetSpecify=off  PositionTargetPriority=High  PositionTargetValue=0  PositionTargetValueUnits=m  VelocityTargetSpecify=off  VelocityTargetPriority=High  VelocityTargetValue=0  VelocityTargetValueUnits=m/s  EquilibriumPosition=0  EquilibriumPositionUnits=m  SpringStiffness=0  SpringStiffnessUnits=N/m  DampingCoefficient=0  DampingCoefficientUnits=N/(m/s)  LowerLimitSpecify=on  LowerLimitBound=-0.5*strokeYMax  LowerLimitBoundUnits=m  LowerLimitStiffness=1e6  LowerLimitStiffnessUnits=N/m  LowerLimitDamping=1e3  LowerLimitDampingUnits=N/(m/s)  LowerLimitTransitionRegionWidth=1e-4  LowerLimitTransitionRegionWidthUnits=m  UpperLimitSpecify=on  UpperLimitBound=0.5*strokeYMax  UpperLimitBoundUnits=m  UpperLimitStiffness=1e6  UpperLimitStiffnessUnits=N/m  UpperLimitDamping=1e3  UpperLimitDampingUnits=N/(m/s)  UpperLimitTransitionRegionWidth=1e-4  UpperLimitTransitionRegionWidthUnits=m  TorqueActuationMode=InputTorque  MotionActuationMode=ComputedMotion  SensePosition=on  SenseVelocity=on  SenseAcceleration=on  SenseTorqueForce=off  SenseLowerLimitTorqueForce=off  SenseUpperLimitTorqueForce=off
  Rigid Transform1 : sm_lib/Frames and Transforms/Rigid Transform  RotationMethod=None  FollAlignAxisA=+X  BaseAlignAxisA=+Y  FollAlignAxisB=+Y  BaseAlignAxisB=+Z  RotationStandardAxis=+Z  RotationAngle=0  RotationAngleUnits=deg  RotationArbitraryAxis=[0 0 1]  RotationSequenceAxes=BaseAxes  RotationSequence=XYZ  RotationSequenceAngles=[0 0 0]  RotationSequenceAnglesUnits=deg  RotationMatrix=[1 0 0;0 1 0;0 0 1]  Quaternion=[1 0 0 0]  TranslationMethod=StandardAxis  TranslationCartesianOffset=[0 0 0]  TranslationCartesianOffsetUnits=m  TranslationStandardAxis=+Y  TranslationStandardOffset=-positionColumn1(2)  TranslationStandardOffsetUnits=m  TranslationROffset=0  TranslationROffsetUnits=m  TranslationThetaOffset=0  TranslationThetaOffsetUnits=deg  TranslationZOffset=0  TranslationZOffsetUnits=m
  Rigid Transform3 : sm_lib/Frames and Transforms/Rigid Transform  RotationMethod=StandardAxis  FollAlignAxisA=+X  BaseAlignAxisA=+Y  FollAlignAxisB=+Y  BaseAlignAxisB=+Z  RotationStandardAxis=+X  RotationAngle=-90  RotationAngleUnits=deg  RotationArbitraryAxis=[0 0 1]  RotationSequenceAxes=FollowerAxes  RotationSequence=XYX  RotationSequenceAngles=[0 0 0]  RotationSequenceAnglesUnits=deg  RotationMatrix=[1 0 0;0 1 0;0 0 1]  Quaternion=[1 0 0 0]  TranslationMethod=None  TranslationCartesianOffset=[0 0 0]  TranslationCartesianOffsetUnits=m  TranslationStandardAxis=+Z  TranslationStandardOffset=0  TranslationStandardOffsetUnits=m  TranslationROffset=0  TranslationROffsetUnits=m  TranslationThetaOffset=0  TranslationThetaOffsetUnits=deg  TranslationZOffset=0  TranslationZOffsetUnits=m
  Rigid Transform4 : sm_lib/Frames and Transforms/Rigid Transform  RotationMethod=StandardAxis  FollAlignAxisA=+X  BaseAlignAxisA=+Y  FollAlignAxisB=+Y  BaseAlignAxisB=+Z  RotationStandardAxis=+X  RotationAngle=90  RotationAngleUnits=deg  RotationArbitraryAxis=[0 0 1]  RotationSequenceAxes=FollowerAxes  RotationSequence=XYX  RotationSequenceAngles=[0 0 0]  RotationSequenceAnglesUnits=deg  RotationMatrix=[1 0 0;0 1 0;0 0 1]  Quaternion=[1 0 0 0]  TranslationMethod=None  TranslationCartesianOffset=[0 0 0]  TranslationCartesianOffsetUnits=m  TranslationStandardAxis=+Z  TranslationStandardOffset=0  TranslationStandardOffsetUnits=m  TranslationROffset=0  TranslationROffsetUnits=m  TranslationThetaOffset=0  TranslationThetaOffsetUnits=deg  TranslationZOffset=0  TranslationZOffsetUnits=m
  Y-Axis Linear Stage : CartesianLib/Linear Stage  systemGuide=Rail-block  axisGuide=Y-axis  stroke=1  widthRail=0.05  diaScrew=0.05  typeInertiaGuide=Calculate from Geometry  densityGuide=2700  massGuide=0.1  CMGuide=[0 0 0]  MOIGuide=[0.01 0.01 0.01]  POIGuide=[0 0 0]  typeInertiaCarriage=Calculate from Geometry  densityCarriage=2700  massCarriage=0.1  CMCarriage=[0 0 0]  MOICarriage=[0.01 0.01 0.01]  POICarriage=[0 0 0]  colorGuide=colorGuideY  colorCarriage=colorCarriageY
  YA : PMIOPort  Side=Left
  F : PMIOPort  Port=2  Side=Left
  B : PMIOPort  Port=3  Side=Right
  Out Bus Element : Outport  PortName=YS  Element=Yp (m)
  BusElementOut : Outport  PortName=YS  Element=Yv (m/s)
  BusElementOut1 : Outport  PortName=YS  Element=Ya (m^2/s)
  wires:
  PS-Simulink Converter2/1 -> BusElementOut1/1
  PS-Simulink Converter1/1 -> BusElementOut/1
  PS-Simulink Converter/1 -> Out Bus Element/1
  connections:
  Prismatic Joint2/RConn4 -- PS-Simulink Converter2/LConn1
  Prismatic Joint2/RConn3 -- PS-Simulink Converter1/LConn1
  Prismatic Joint2/RConn2 -- PS-Simulink Converter/LConn1
  F/RConn1 -- Y-Axis Linear Stage/LConn1
  Rigid Transform1/LConn1 -- B/RConn1
  Prismatic Joint2/LConn2 -- YA/RConn1
  Rigid Transform1/RConn1 -- Y-Axis Linear Stage/RConn1
  Prismatic Joint2/RConn1 -- Rigid Transform4/LConn1
  Rigid Transform3/LConn1 -- Y-Axis Linear Stage/RConn2
  Rigid Transform4/RConn1 -- Y-Axis Linear Stage/LConn2
  Prismatic Joint2/LConn1 -- Rigid Transform3/RConn1

== system CantileverCartesianRobotSubsystem/CantileverCartesianRobotVariant/XYZ Cartesian/Z-Axis Unit ==
  PS-Simulink Converter : nesl_utility/PS-Simulink Converter  PhysicalDomain=network_engine_domain  SubClassName=ps_output  LeftPortType=input  RightPortType=output  PseudoPeriodic=off  Frequencies=[]  VectorFormat=inherit  Unit=inherit  AffineConversion=off
  PS-Simulink Converter1 : nesl_utility/PS-Simulink Converter  PhysicalDomain=network_engine_domain  SubClassName=ps_output  LeftPortType=input  RightPortType=output  PseudoPeriodic=off  Frequencies=[]  VectorFormat=inherit  Unit=inherit  AffineConversion=off
  PS-Simulink Converter2 : nesl_utility/PS-Simulink Converter  PhysicalDomain=network_engine_domain  SubClassName=ps_output  LeftPortType=input  RightPortType=output  PseudoPeriodic=off  Frequencies=[]  VectorFormat=inherit  Unit=inherit  AffineConversion=off
  Prismatic Joint2 : sm_lib/Joints/Prismatic Joint  JointMode=Normal  CompositeWrenchDir=FollowerOnBase  CompositeWrenchFrame=BaseFrame  SenseConstraintForce=off  SenseConstraintTorque=off  SenseTotalForce=off  SenseTotalTorque=off  PositionTargetSpecify=off  PositionTargetPriority=High  PositionTargetValue=0  PositionTargetValueUnits=m  VelocityTargetSpecify=off  VelocityTargetPriority=High  VelocityTargetValue=0  VelocityTargetValueUnits=m/s  EquilibriumPosition=0  EquilibriumPositionUnits=m  SpringStiffness=0  SpringStiffnessUnits=N/m  DampingCoefficient=0  DampingCoefficientUnits=N/(m/s)  LowerLimitSpecify=on  LowerLimitBound=-0.5*strokeZMax  LowerLimitBoundUnits=m  LowerLimitStiffness=1e6  LowerLimitStiffnessUnits=N/m  LowerLimitDamping=1e3  LowerLimitDampingUnits=N/(m/s)  LowerLimitTransitionRegionWidth=1e-4  LowerLimitTransitionRegionWidthUnits=m  UpperLimitSpecify=on  UpperLimitBound=0.5*strokeZMax  UpperLimitBoundUnits=m  UpperLimitStiffness=1e6  UpperLimitStiffnessUnits=N/m  UpperLimitDamping=1e3  UpperLimitDampingUnits=N/(m/s)  UpperLimitTransitionRegionWidth=1e-4  UpperLimitTransitionRegionWidthUnits=m  TorqueActuationMode=InputTorque  MotionActuationMode=ComputedMotion  SensePosition=on  SenseVelocity=on  SenseAcceleration=on  SenseTorqueForce=off  SenseLowerLimitTorqueForce=off  SenseUpperLimitTorqueForce=off
  Rigid Transform1 : sm_lib/Frames and Transforms/Rigid Transform  RotationMethod=None  FollAlignAxisA=+X  BaseAlignAxisA=+Y  FollAlignAxisB=+Y  BaseAlignAxisB=+Z  RotationStandardAxis=+Z  RotationAngle=0  RotationAngleUnits=deg  RotationArbitraryAxis=[0 0 1]  RotationSequenceAxes=BaseAxes  RotationSequence=XYZ  RotationSequenceAngles=[0 0 0]  RotationSequenceAnglesUnits=deg  RotationMatrix=[1 0 0;0 1 0;0 0 1]  Quaternion=[1 0 0 0]  TranslationMethod=StandardAxis  TranslationCartesianOffset=[0 0 0]  TranslationCartesianOffsetUnits=m  TranslationStandardAxis=+Z  TranslationStandardOffset=shiftZAxisDown  TranslationStandardOffsetUnits=m  TranslationROffset=0  TranslationROffsetUnits=m  TranslationThetaOffset=0  TranslationThetaOffsetUnits=deg  TranslationZOffset=0  TranslationZOffsetUnits=m
  Rigid Transform2 : sm_lib/Frames and Transforms/Rigid Transform  RotationMethod=None  FollAlignAxisA=+X  BaseAlignAxisA=+Y  FollAlignAxisB=+Y  BaseAlignAxisB=+Z  RotationStandardAxis=+X  RotationAngle=0  RotationAngleUnits=deg  RotationArbitraryAxis=[0 0 1]  RotationSequenceAxes=FollowerAxes  RotationSequence=XYX  RotationSequenceAngles=[0 0 0]  RotationSequenceAnglesUnits=deg  RotationMatrix=[1 0 0;0 1 0;0 0 1]  Quaternion=[1 0 0 0]  TranslationMethod=None  TranslationCartesianOffset=[0 0 0]  TranslationCartesianOffsetUnits=m  TranslationStandardAxis=+Z  TranslationStandardOffset=0  TranslationStandardOffsetUnits=m  TranslationROffset=0  TranslationROffsetUnits=m  TranslationThetaOffset=0  TranslationThetaOffsetUnits=deg  TranslationZOffset=0  TranslationZOffsetUnits=m
  Rigid Transform3 : sm_lib/Frames and Transforms/Rigid Transform  RotationMethod=None  FollAlignAxisA=+X  BaseAlignAxisA=+Y  FollAlignAxisB=+Y  BaseAlignAxisB=+Z  RotationStandardAxis=+X  RotationAngle=0  RotationAngleUnits=deg  RotationArbitraryAxis=[0 0 1]  RotationSequenceAxes=FollowerAxes  RotationSequence=XYX  RotationSequenceAngles=[0 0 0]  RotationSequenceAnglesUnits=deg  RotationMatrix=[1 0 0;0 1 0;0 0 1]  Quaternion=[1 0 0 0]  TranslationMethod=None  TranslationCartesianOffset=[0 0 0]  TranslationCartesianOffsetUnits=m  TranslationStandardAxis=+Z  TranslationStandardOffset=0  TranslationStandardOffsetUnits=m  TranslationROffset=0  TranslationROffsetUnits=m  TranslationThetaOffset=0  TranslationThetaOffsetUnits=deg  TranslationZOffset=0  TranslationZOffsetUnits=m
  Z-Axis Linear Stage : CartesianLib/Linear Stage  systemGuide=Rail-block  axisGuide=Z-axis  stroke=1  widthRail=0.05  diaScrew=0.05  typeInertiaGuide=Calculate from Geometry  densityGuide=2700  massGuide=0.1  CMGuide=[0 0 0]  MOIGuide=[0.01 0.01 0.01]  POIGuide=[0 0 0]  typeInertiaCarriage=Calculate from Geometry  densityCarriage=2700  massCarriage=0.1  CMCarriage=[0 0 0]  MOICarriage=[0.01 0.01 0.01]  POICarriage=[0 0 0]  colorGuide=colorGuideZ  colorCarriage=colorCarriageZ
  ZA : PMIOPort  Side=Left
  F : PMIOPort  Port=2  Side=Left
  B : PMIOPort  Port=3  Side=Right
  Out Bus Element : Outport  PortName=ZS  Element=Zp (m)
  BusElementOut : Outport  PortName=ZS  Element=Zv (m/s)
  BusElementOut1 : Outport  PortName=ZS  Element=Za (m^2/s)
  wires:
  PS-Simulink Converter2/1 -> BusElementOut1/1
  PS-Simulink Converter1/1 -> BusElementOut/1
  PS-Simulink Converter/1 -> Out Bus Element/1
  connections:
  Prismatic Joint2/RConn4 -- PS-Simulink Converter2/LConn1
  Prismatic Joint2/RConn3 -- PS-Simulink Converter1/LConn1
  Prismatic Joint2/RConn2 -- PS-Simulink Converter/LConn1
  F/RConn1 -- Z-Axis Linear Stage/LConn1
  Rigid Transform1/LConn1 -- B/RConn1
  Prismatic Joint2/LConn2 -- ZA/RConn1
  Rigid Transform1/RConn1 -- Z-Axis Linear Stage/RConn1
  Prismatic Joint2/RConn1 -- Rigid Transform3/LConn1
  Rigid Transform2/LConn1 -- Z-Axis Linear Stage/RConn2
  Rigid Transform3/RConn1 -- Z-Axis Linear Stage/LConn2
  Prismatic Joint2/LConn1 -- Rigid Transform2/RConn1
